simulink model "sysgenDWT"  (Simulink 7.0)
settings: Solver=ode45  StartTime=0.0  StopTime=4096+1024+100  RelTol=1e-3
PreLoadFcn:
  | xlrequire('imageData.mat'); xlrequire('PreLoadFcn');
PostLoadFcn:
  | open_system('sysgenDWT/Processor/Memory Controller','force'); pause(0.50); open_system('sysgenDWT');pause(0.50); close_system('sysgenDWT/Processor/Memory Controller');pause(0.50); close_system('sysgenDWT/Processor');
StopFcn:
  | xlrequire('StopFcn');
values from neighbouring files (symbols this model uses):
  b1Init = sysgenDWT_imageData( stride + dither )    [sysgenDWT_PreLoadFcn.m]
  b2Init = sysgenDWT_imageData( stride + not(dither) )    [sysgenDWT_PreLoadFcn.m]
libraries: xbsIndex_r4 x214, dspindex x4, dspmtrx3 x4, dspsnks4 x3, xbsCopyrightNotice_r4 x1, dspsrcs4 x1
(part 3 of 3)

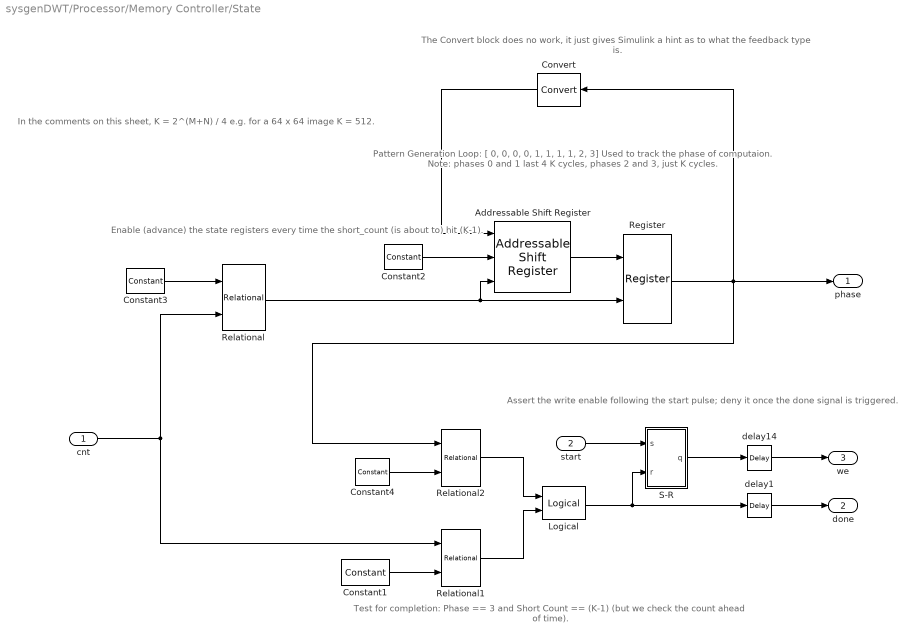
== system sysgenDWT/Processor/Memory Controller/State ==
  note: Pattern Generation Loop:
      | [ 0, 0, 0, 0, 1, 1, 1, 1, 2, 3]
      | Used to track the phase of computaion.
      | Note: phases 0 and 1 last 4 K cycles,
      | phases 2 and 3, just K cycles.
  note: Test for completion:
      | Phase == 3  and
      | Short Count == (K-1)
      | (but we check the count ahead of time).
  note: Enable (advance) the
      | state registers every time
      | the short_count (is about to)
      | hit  (K-1).
  note: Assert the write enable following
      | the start pulse;  deny it once the
      | done signal is triggered.
  note: In the comments on this sheet,
      |  K = 2^(M+N) / 4
      | e.g. for a 64 x 64 image K = 512.
  note: The Convert block does no work, it  just gives
      | Simulink a hint as to what the feedback type is.
  cnt : Inport  OutDataType=sfix(16)  OutScaling=2^0
  start : Inport  Port=2  OutDataType=sfix(16)  OutScaling=2^0
  Addressable Shift Register : xbsIndex_r4/Addressable Shift Register  infer_latency=on  depth=2  initVector=[3 2 1 1 1 1 0 0 0]  en=on  dbl_ovrd=off  use_behavioral_HDL=off  use_rpm=off  block_type=addrsr
      settings: infoedit="Delay of configurable length.  Any element in the delay line can be addressed and driven onto the output port.<P><P>Hardware notes: Implemented using SRL16s.  If a Virtex-II device is used, multiple SRLC16s are cascaded together."  xl_area=[1 0 0 2 0 0 0]  block_version=VER_STRING_GOES_HERE
  Constant1 : xbsIndex_r4/Constant  arith_type=Unsigned  const=power(2,M+N-2) - 4  n_bits=M+N-3  bin_pt=0  explicit_period=off  period=1  equ=P=C  opselect=C  inp2=PCIN>>17  opr=+  inp1=P  carry=CIN  dbl_ovrd=off  block_type=constant
      settings: block_version=VER_STRING_GOES_HERE
  Constant2 : xbsIndex_r4/Constant  arith_type=Unsigned  const=8  n_bits=4  bin_pt=0  explicit_period=off  period=1  equ=P=C  opselect=C  inp2=PCIN>>17  opr=+  inp1=P  carry=CIN  dbl_ovrd=off  block_type=constant
      settings: block_version=VER_STRING_GOES_HERE
  Constant3 : xbsIndex_r4/Constant  arith_type=Unsigned  const=power(2,M+N-2) - 2  n_bits=M+N-3  bin_pt=0  explicit_period=off  period=1  equ=P=C  opselect=C  inp2=PCIN>>17  opr=+  inp1=P  carry=CIN  dbl_ovrd=off  block_type=constant
      settings: block_version=VER_STRING_GOES_HERE
  Constant4 : xbsIndex_r4/Constant  arith_type=Unsigned  const=3  n_bits=2  bin_pt=0  explicit_period=off  period=1  equ=P=C  opselect=C  inp2=PCIN>>17  opr=+  inp1=P  carry=CIN  dbl_ovrd=off  block_type=constant
      settings: block_version=VER_STRING_GOES_HERE
  Convert : xbsIndex_r4/Convert  Orientation=left  arith_type=Unsigned  n_bits=2  bin_pt=0  quantization=Truncate  overflow=Wrap  latency=0  dbl_ovrd=off  pipeline=off  block_type=convert
      settings: infoedit=The input is presented at the output after quantization and overflow effects.<P><P>Hardware notes: Additional hardware is used when rounding or saturation is selected and output width is less than the input width.  xl_area=[0 0 0 0 0 0 0]  block_version=VER_STRING_GOES_HERE
  Logical : xbsIndex_r4/Logical  logical_function=AND  inputs=2  en=off  latency=0  precision=Full  arith_type=Unsigned  n_bits=8  bin_pt=2  align_bp=on  dbl_ovrd=off  block_type=logical
      settings: xl_area=[1 0 0 1 0 0 0]  block_version=VER_STRING_GOES_HERE
  Register : xbsIndex_r4/Register  init=0  rst=off  en=on  dbl_ovrd=off  block_type=register
      settings: xl_area=[1 2 0 0 0 0 0]  block_version=VER_STRING_GOES_HERE
  Relational : xbsIndex_r4/Relational  mode=a=b  en=off  latency=1  dbl_ovrd=off  block_type=relational
      settings: xl_area=[3 1 0 5 0 0 0]  block_version=VER_STRING_GOES_HERE
  Relational1 : xbsIndex_r4/Relational  mode=a=b  en=off  latency=2  dbl_ovrd=off  block_type=relational
      settings: xl_area=[3 2 0 5 0 0 0]  block_version=VER_STRING_GOES_HERE
  Relational2 : xbsIndex_r4/Relational  mode=a=b  en=off  latency=2  dbl_ovrd=off  block_type=relational
      settings: xl_area=[1 2 0 1 0 0 0]  block_version=VER_STRING_GOES_HERE
  S-R : Subsystem
  delay1 : xbsIndex_r4/Delay  en=off  latency=2  dbl_ovrd=off  reg_retiming=off  block_type=delay
      settings: infoedit="Delay line having  configurable length.<P><P>Hardware notes: A delay line is a chain, each link of which is an SRL16 followed by a flip-flop. If register retiming is enabled, the delay line is a chain of flip-flops."  xl_area=[1 1 0 1 0 0 0]  block_version=VER_STRING_GOES_HERE
  delay14 : xbsIndex_r4/Delay  en=off  latency=1  dbl_ovrd=off  reg_retiming=off  block_type=delay
      settings: infoedit="Delay line having  configurable length.<P><P>Hardware notes: A delay line is a chain, each link of which is an SRL16 followed by a flip-flop. If register retiming is enabled, the delay line is a chain of flip-flops."  xl_area=[1 1 0 0 0 0 0]  block_version=VER_STRING_GOES_HERE
  phase : Outport  OutDataType=sfix(16)  OutScaling=2^0
  done : Outport  Port=2  OutDataType=sfix(16)  OutScaling=2^0
  we : Outport  Port=3  OutDataType=sfix(16)  OutScaling=2^0
  wires:
  Relational/1 -> Addressable Shift Register/3, Register/2
  Register/1 -> phase/1, Convert/1, Relational2/1
  S-R/1(q) -> delay14/1
  start/1 -> S-R/1(s)
  Constant4/1 -> Relational2/2
  Logical/1 -> S-R/2(r), delay1/1
  delay14/1 -> we/1
  Convert/1 -> Addressable Shift Register/1
  delay1/1 -> done/1
  Constant3/1 -> Relational/1
  cnt/1 -> Relational/2, Relational1/1
  Relational2/1 -> Logical/1
  Relational1/1 -> Logical/2
  Constant1/1 -> Relational1/2
  Constant2/1 -> Addressable Shift Register/2
  Addressable Shift Register/1 -> Register/1

== system sysgenDWT/Processor/Memory Controller/State/S-R ==
  note: 1-bit register used as Set-Reset Flip Flop.
  s : Inport  OutDataType=sfix(16)  OutScaling=2^0
  r : Inport  Port=2  OutDataType=sfix(16)  OutScaling=2^0
  Register2 : xbsIndex_r4/Register  init=0  rst=on  en=on  dbl_ovrd=off  block_type=register
      settings: xl_area=[1 1 0 0 0 0 0]  block_version=VER_STRING_GOES_HERE
  q : Outport  OutDataType=sfix(16)  OutScaling=2^0
  wires:
  s/1 -> Register2/1, Register2/3
  r/1 -> Register2/2
  Register2/1 -> q/1
